simulink model "DESIG_analysis"  (R2025b)
settings: Solver=ode1  StartTime=0.0  StopTime=Tf  FixedStep=Tstep  RelTol=1e-3
values from neighbouring files (symbols this model uses):
  Kd = (2*W_cl*Zeta_cl*Time_const - 1)/Km    [DESIG_mat.m]    (also in Designation.m)
  Km = 11.8676/ 12.6778    (= 0.936093012983)    [DESIG_mat.m]    (also in Designation.m; Designation_mat.m = 1.00750476048)
  Kp = (Time_const/Km)*W_cl^2    (= 66.0622198254)    [DESIG_mat.m]    (also in Designation.m = 97.4080690283)
  sim_deadZone = 20.0 * scaler_deg2rad    (= 0.349065850399)    [DESIG_mat.m]
  sim_saturation = 1300 * scaler_deg2rad    (= 22.6892802759)    [DESIG_mat.m]
  Time_const = 1 / 12.6778    (= 0.0788780387764)    [DESIG_mat.m]    (also in Designation.m; Designation_mat.m = 0.0933427920696)
  Tsample = 0.005    [DESIG_mat.m]    (also in Designation.m; Designation_mat.m)
settings Model: Creator=GILBERT  LastModifiedBy=GILBERT

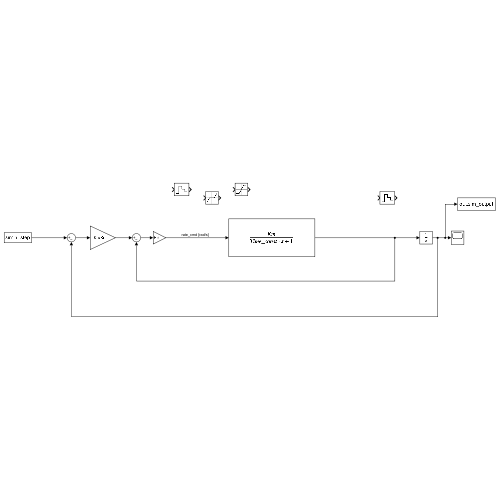
[thumbnail: Simulink's stored preview of the top-level diagram]
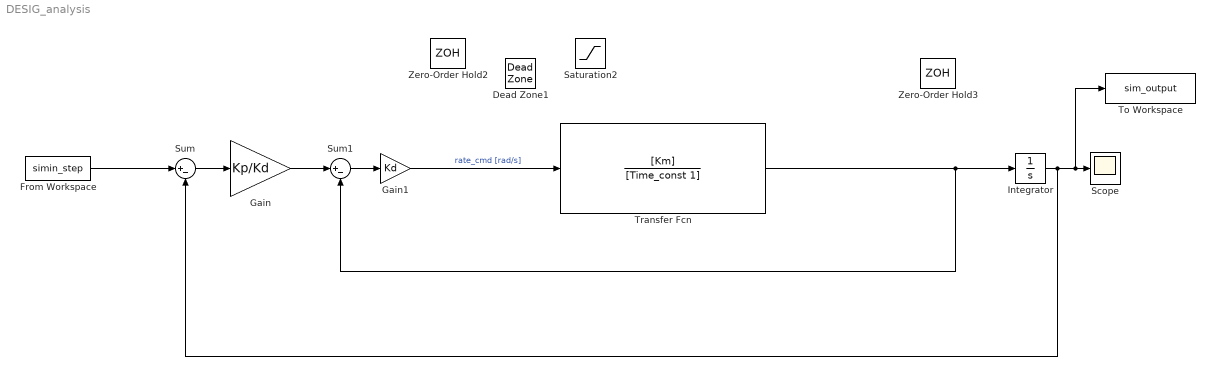
== system DESIG_analysis ==
  Dead Zone1 : DeadZone  LowerValue=- sim_deadZone  UpperValue=sim_deadZone
  From Workspace : FromWorkspace  VariableName=simin_step
  Gain : Gain  Gain=Kp/Kd
  Gain1 : Gain  Gain=Kd
  Integrator : Integrator
  Saturation2 : Saturate  UpperLimit=sim_saturation  LowerLimit=-sim_saturation
  Scope : Scope
      settings: ActiveDisplayYMinimum=-3.9120434137934068  ActiveDisplayYMaximum=35.208390724140671
  Sum : Sum  Inputs=|+-
  Sum1 : Sum  Inputs=|+-
  To Workspace : ToWorkspace  VariableName=sim_output  SampleTime=-1
  Transfer Fcn : TransferFcn  Numerator=[Km]  Denominator=[Time_const 1]
  Zero-Order Hold2 : ZeroOrderHold  SampleTime=Tsample
  Zero-Order Hold3 : ZeroOrderHold  SampleTime=Tsample
  wires:
  Sum/1 -> Gain/1
  Gain/1 -> Sum1/1
  Sum1/1 -> Gain1/1
  Integrator/1 -> To Workspace/1, Scope/1, Sum/2
  Transfer Fcn/1 -> Sum1/2, Integrator/1
  From Workspace/1 -> Sum/1
  Gain1/1 -> Transfer Fcn/1  "rate_cmd [rad/s]"
